simulink model "SEPIC_hybrid_closed_loop"  (R2020a)
settings: Solver=FixedStepAuto  StartTime=0.0  StopTime=0.05  FixedStep=Ts  RelTol=1e-8
values from neighbouring files (symbols this model uses):
  E = 300    [parameters_SEPIC.m]    (also in test_sepic_1.m = @(t) 300)
  L1 = 2.57e-3    (= 0.00257)    [parameters_SEPIC.m]
  L2 = 1.71e-3    (= 0.00171)    [parameters_SEPIC.m]
  R = 80    [parameters_SEPIC.m]    (also in test_boost_1.m = @(t) (t <= tfin/2)*12 + (t>tfin/2)*15; test_sepic_1.m = @(t) 80)
  rC1 = 350e-3    (= 0.35)    [parameters_SEPIC.m]
  rC2 = 270e-3    (= 0.27)    [parameters_SEPIC.m]
  rDS1 = 0.01    [parameters_SEPIC.m]
  rDS2 = 80e-3    (= 0.08)    [parameters_SEPIC.m]
  Ts = 1/fPWM/100    (= 1e-07)    [parameters_SEPIC.m]
  VF1 = 0.2    [parameters_SEPIC.m]
  VF2 = 0.62    [parameters_SEPIC.m]
undefined symbols (not defined in the file or in its folder): Down, Ks, Up
libraries: fl_lib x13, nesl_utility x12, ee_lib x4, simulink x2, eePwmGenerator x1
settings Model: Creator=Vlad  LastModifiedBy=mircea
settings SFSimCC: CustomCodeUndefinedFunction=UseInterfaceOnly

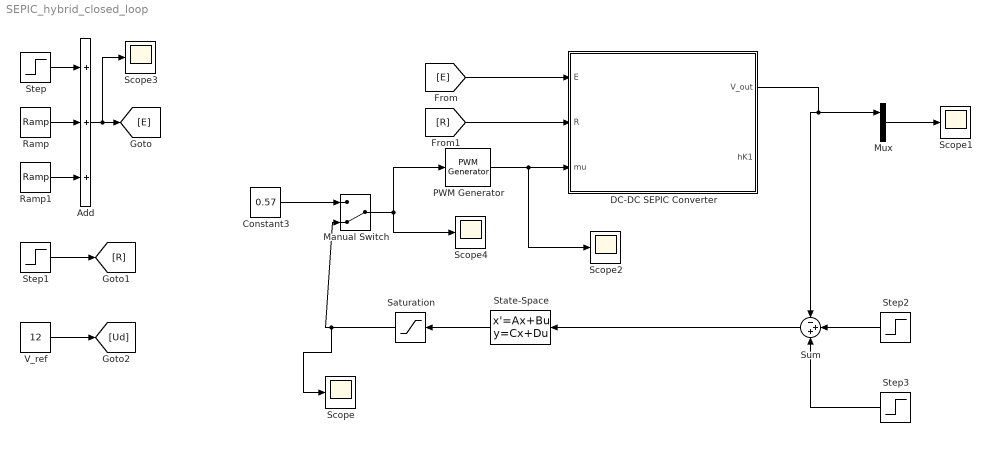
== system SEPIC_hybrid_closed_loop ==
  Add : Sum  Inputs=+++
  Constant3 : Constant  Value=0.57
  DC-DC SEPIC Converter : Subsystem
  Manual Switch : ManualSwitch  CurrentSetting=0
  Mux : Mux  Inputs=2
  PWM Generator : eePwmGenerator/PWM Generator  CarrCount=Up-Down  Tper=TPWM  Ts=Ts
  Ramp : simulink/Sources/Ramp  slope=30  start=0.2  InitialOutput=0
  Ramp1 : simulink/Sources/Ramp  slope=-60  start=0.3  InitialOutput=0
  Saturation : Saturate  UpperLimit=0.95  LowerLimit=0
  Scope{,1..4} (5 alike) : Scope
  State-Space : StateSpace  A=Ks.A  B=Ks.B  C=Ks.C  D=Ks.D  InitialCondition=0
  Step : Step  Time=0.1  Before=E  After=1.2*E  SampleTime=0
  Step1 : Step  Time=0.15  Before=R  After=1.2*R  SampleTime=0
  Step2 : Step  Time=0.01  Before=380  After=400  SampleTime=0
  Step3 : Step  Time=0.025  After=20  SampleTime=0
  Sum : Sum  Inputs=-++
  V_ref : Constant  Value=12
  wires:
  V_ref/1 -> [Ud]
  Step1/1 -> [R]
  Ramp1/1 -> Add/3
  Ramp/1 -> Add/2
  Step/1 -> Add/1
  Add/1 -> Scope3/1, [E]
  [R] -> DC-DC SEPIC Converter/2(R)
  [E] -> DC-DC SEPIC Converter/1(E)
  Constant3/1 -> Manual Switch/1
  Manual Switch/1 -> Scope4/1, PWM Generator/1
  Mux/1 -> Scope1/1
  DC-DC SEPIC Converter/1(V_out) -> Sum/1, Mux/1
  PWM Generator/1 -> Scope2/1, DC-DC SEPIC Converter/3(mu)
  Step2/1 -> Sum/2
  Sum/1 -> State-Space/1
  State-Space/1 -> Saturation/1
  Saturation/1 -> Scope/1, Manual Switch/2
  Step3/1 -> Sum/3

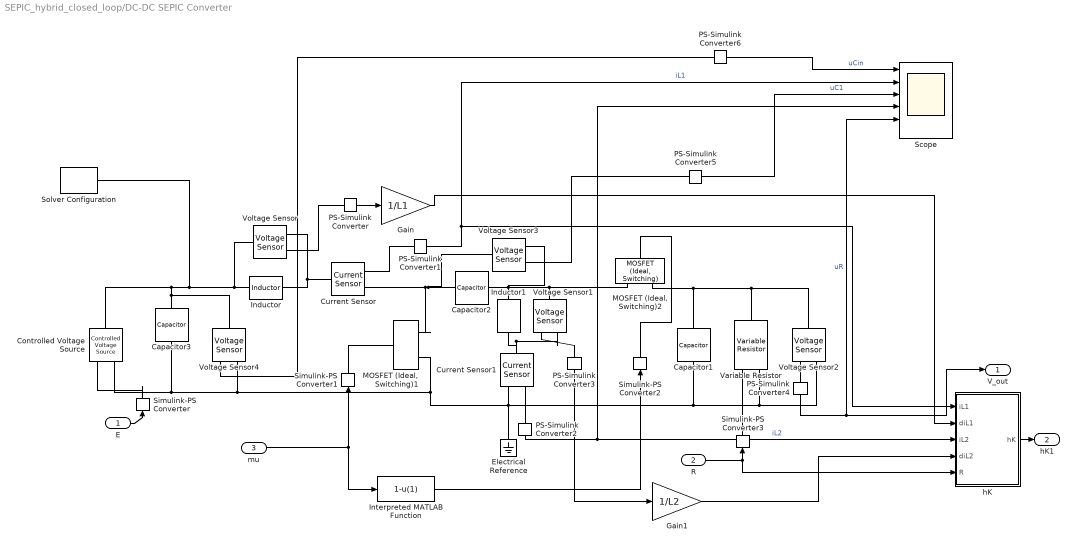
== system SEPIC_hybrid_closed_loop/DC-DC SEPIC Converter ==
  E : Inport
  R : Inport  Port=2
  mu : Inport  Port=3
  Capacitor1 : fl_lib/Electrical/Electrical Elements/Capacitor  c=C2 F  r=rC2 Ohm  g=0 1/Ohm  i_specify=off  i_priority=None  i=0 A  i_nominal_specify=off  i_nominal_unit=A  i_nominal_value=1  v_specify=on  v_priority=None  v=uC20 V  v_nominal_specify=off  v_nominal_unit=V  v_nominal_value=1  vc_specify=off  vc_priority=High  vc=0 V  vc_nominal_specify=off  vc_nominal_unit=V  vc_nominal_value=1
  Capacitor2 : fl_lib/Electrical/Electrical Elements/Capacitor  c=C1 F  r=rC1 Ohm  g=0 1/Ohm  i_specify=off  i_priority=None  i=0 A  i_nominal_specify=off  i_nominal_unit=A  i_nominal_value=1  v_specify=on  v_priority=None  v=uC10 V  v_nominal_specify=off  v_nominal_unit=V  v_nominal_value=1  vc_specify=off  vc_priority=High  vc=0 V  vc_nominal_specify=off  vc_nominal_unit=V  vc_nominal_value=1
  Capacitor3 : fl_lib/Electrical/Electrical Elements/Capacitor  c=Cin F  r=rCin Ohm  g=0 1/Ohm  i_specify=off  i_priority=None  i=0 A  i_nominal_specify=off  i_nominal_unit=A  i_nominal_value=1  v_specify=on  v_priority=None  v=uCin0 V  v_nominal_specify=off  v_nominal_unit=V  v_nominal_value=1  vc_specify=off  vc_priority=High  vc=0 V  vc_nominal_specify=off  vc_nominal_unit=V  vc_nominal_value=1
  Controlled Voltage Source : fl_lib/Electrical/Electrical Sources/Controlled Voltage Source
  Current Sensor : fl_lib/Electrical/Electrical Sensors/Current Sensor
  Current Sensor1 : fl_lib/Electrical/Electrical Sensors/Current Sensor
  Electrical Reference : fl_lib/Electrical/Electrical Elements/Electrical Reference
  Gain : Gain  Gain=1/L1
  Gain1 : Gain  Gain=1/L2
  Inductor : ee_lib/Passive/Inductor  l=L1 H  L_tol=20  enable_L_tol=0  tol_distribution=1  nSigma=4  r=rL1 Ohm  g=0 1/Ohm  enable_operating_limits=0  operating_limit_action=2  max_working_current=1 A  power_rating=1 W  enable_faults=0  fault_action=1  lambdaPercent=50  k_faulted=0.9999  turnsShort=0  openCct=0  groundShort=0  groundShortG=0 1/Ohm  tau_fault=1e-3 s  enable_temporal_fault=0  t_fault=1 s  enable_behavioral_fault=0  max_permissible_voltage=100 V  n_fail_on_voltage=1  max_permissible_current=1 A  t_fail_on_current=1 s  i_L_specify=on  i_L_priority=High  i_L=iL10 A  i_L_nominal_specify=off  i_L_nominal_unit=A  i_L_nominal_value=1
  Inductor1 : ee_lib/Passive/Inductor  l=L2 H  L_tol=20  enable_L_tol=0  tol_distribution=1  nSigma=4  r=rL2 Ohm  g=0 1/Ohm  enable_operating_limits=0  operating_limit_action=2  max_working_current=1 A  power_rating=1 W  enable_faults=0  fault_action=1  lambdaPercent=50  k_faulted=0.9999  turnsShort=0  openCct=0  groundShort=0  groundShortG=0 1/Ohm  tau_fault=1e-3 s  enable_temporal_fault=0  t_fault=1 s  enable_behavioral_fault=0  max_permissible_voltage=100 V  n_fail_on_voltage=1  max_permissible_current=1 A  t_fail_on_current=1 s  i_L_specify=on  i_L_priority=High  i_L=iL20 A  i_L_nominal_specify=off  i_L_nominal_unit=A  i_L_nominal_value=1
  Interpreted MATLAB Function : MATLABFcn  MATLABFcn=1-u(1)
  "MOSFET (Ideal, Switching)1" : ee_lib/Semiconductors & Converters/MOSFET (Ideal, Switching)  Rds=rDS1 Ohm  Goff=1e-6 1/Ohm  Vth=0.5 V  diode_param=2  diode_Vf=VF1 V  diode_Ron=0.001 Ohm  diode_Goff=1e-5 1/Ohm  diode_C=50e-9 F  diode_iRM=-235 A  diode_iF=300 A  diode_idot=-50 A/us  diode_trr_param=1  diode_trr_factor=3  diode_trr=15 us  diode_Qrr=1500 s*uA  thermal_loss_option=ee.enum.converters.thermalLossOption.constantvalues  Voff=300 V  Tau=1e-4 s  Tj=[298.15, 398.15] K  Iout_scalar=600 A  Eon_scalar=22.86e-3 J  Eoff_scalar=17.14e-3 J  Von_scalar=2.7 V  Iout_data=[0, 10, 50, 100, 200, 400, 600] A  Eon_data=[0, .29, 1.43, 2.86, 5.71, 13.14, 22.86; 0, .57, 2.63, 5.14, 10.29, 20.57, 30.29] * 1e-3 J  Eoff_data=[0, .21, 1.07, 2.14, 4.29, 9.86, 17.14; 0, .43, 1.97, 3.86, 7.71, 15.43, 22.71] * 1e-3 J  Von_data=[0, 1.1, 1.3, 1.45, 1.75, 2.25, 2.7; 0, 1, 1.15, 1.35, 1.7, 2.35, 3] V
  "MOSFET (Ideal, Switching)2" : ee_lib/Semiconductors & Converters/MOSFET (Ideal, Switching)  Rds=rDS2 Ohm  Goff=1e-6 1/Ohm  Vth=0.5 V  diode_param=2  diode_Vf=VF2 V  diode_Ron=0.001 Ohm  diode_Goff=1e-5 1/Ohm  diode_C=50e-9 F  diode_iRM=-235 A  diode_iF=300 A  diode_idot=-50 A/us  diode_trr_param=1  diode_trr_factor=3  diode_trr=15 us  diode_Qrr=1500 s*uA  thermal_loss_option=ee.enum.converters.thermalLossOption.constantvalues  Voff=300 V  Tau=1e-4 s  Tj=[298.15, 398.15] K  Iout_scalar=600 A  Eon_scalar=22.86e-3 J  Eoff_scalar=17.14e-3 J  Von_scalar=2.7 V  Iout_data=[0, 10, 50, 100, 200, 400, 600] A  Eon_data=[0, .29, 1.43, 2.86, 5.71, 13.14, 22.86; 0, .57, 2.63, 5.14, 10.29, 20.57, 30.29] * 1e-3 J  Eoff_data=[0, .21, 1.07, 2.14, 4.29, 9.86, 17.14; 0, .43, 1.97, 3.86, 7.71, 15.43, 22.71] * 1e-3 J  Von_data=[0, 1.1, 1.3, 1.45, 1.75, 2.25, 2.7; 0, 1, 1.15, 1.35, 1.7, 2.35, 3] V
  PS-Simulink Converter{,1..6} (7 alike) : nesl_utility/PS-Simulink Converter  PhysicalDomain=network_engine_domain  SubClassName=ps_output  LeftPortType=input  RightPortType=output  PseudoPeriodic=off  Frequencies=[]  Unit=inherit  AffineConversion=off
  Scope : Scope  NumInputPorts=6
  Simulink-PS Converter{,1..3} (4 alike) : nesl_utility/Simulink-PS Converter  PhysicalDomain=network_engine_domain  SubClassName=ps_input  LeftPortType=input  RightPortType=output  PseudoPeriodic=off  Frequencies=[]  NoiseDistribution=none  NoiseParameters=[]  Unit=1  AffineConversion=off  FilteringAndDerivatives=provide  SimscapeFilterOrder=1  InputFilterTimeConstant=0.001  UdotUserProvided=0
  Solver Configuration : nesl_utility/Solver Configuration  PhysicalDomain=network_engine_domain  SubClassName=solver  LeftPortType=input  RightPortType=generic  Tones=[]  Harmonics=[]  SimulateNoise=off  Profile=off  UseLocalSampling=off  EnableSwitchedLinearOptims=on  FrequencyDomain=off  UseCCode=off  RelTol=0.001  AbsTol=1e-06  MinStep=1e-09  ToWorkspace=off  RevertToSquareIcSolve=off  NumHomotopyIterations=100  PhasorMode=off  PhasorModeNumHarmonics=1  DoDC=off  ResidualTolerance=1e-09  UseLocalSolver=on  LocalSolverChoice=NE_TRAPEZOIDAL_ADVANCER  LocalSolverSampleTime=Ts  DoFixedCost=off  MaxNonlinIter=3  MaxModeIter=2  LinearAlgebra=auto  EquationFormulation=NE_TIME_EF  DelaysMemoryBudget=1024  AutomaticFiltering=on  FilteringTimeConstant=0.001  PartitionStorageMethod=AS_NEEDED  PartitionMemoryBudget=1024  PartitionMethod=ROBUST
  Variable Resistor : fl_lib/Electrical/Electrical Elements/Variable Resistor  Rmin=0 Ohm  i_specify=off  i_priority=None  i=0 A  i_nominal_specify=off  i_nominal_unit=A  i_nominal_value=1  v_specify=off  v_priority=None  v=0 V  v_nominal_specify=off  v_nominal_unit=V  v_nominal_value=1
  Voltage Sensor{,1..4} (5 alike) : fl_lib/Electrical/Electrical Sensors/Voltage Sensor
  hK : Subsystem
  V_out : Outport
  hK1 : Outport  Port=2
  wires:
  E/1 -> Simulink-PS Converter/1
  Interpreted MATLAB Function/1 -> Simulink-PS Converter2/1
  Gain1/1 -> hK/4(diL2)
  PS-Simulink Converter2/1 -> Scope/4, hK/3(iL2)  "iL2"
  PS-Simulink Converter/1 -> Gain/1
  Gain/1 -> hK/2(diL1)
  R/1 -> hK/5(R), Simulink-PS Converter3/1
  PS-Simulink Converter3/1 -> Gain1/1
  PS-Simulink Converter1/1 -> Scope/2, hK/1(iL1)  "iL1"
  mu/1 -> Simulink-PS Converter1/1, Interpreted MATLAB Function/1
  PS-Simulink Converter4/1 -> Scope/5, V_out/1  "uR"
  hK/1(hK) -> hK1/1
  PS-Simulink Converter5/1 -> Scope/3  "uC1"
  PS-Simulink Converter6/1 -> Scope/1  "uCin"
  connections:
  Inductor1/LConn1 -- Voltage Sensor3/RConn2 -- "MOSFET (Ideal, Switching)2"/RConn2 -- Voltage Sensor1/LConn1 -- Capacitor2/RConn1
  Controlled Voltage Source/LConn1 -- Voltage Sensor4/LConn1 -- Capacitor3/LConn1 -- Solver Configuration/RConn1 -- Voltage Sensor/LConn1 -- Inductor/LConn1
  PS-Simulink Converter4/LConn1 -- Voltage Sensor2/RConn1
  Current Sensor1/LConn1 -- Voltage Sensor1/RConn2 -- Inductor1/RConn1
  Current Sensor/LConn1 -- Voltage Sensor/RConn2 -- Inductor/RConn1
  Capacitor1/LConn1 -- "MOSFET (Ideal, Switching)2"/RConn1 -- Voltage Sensor2/LConn1 -- Variable Resistor/RConn1
  Electrical Reference/LConn1 -- Capacitor3/RConn1 -- Controlled Voltage Source/RConn2 -- Voltage Sensor4/RConn2 -- "MOSFET (Ideal, Switching)1"/RConn2 -- Current Sensor1/RConn2 -- Capacitor1/RConn1 -- Variable Resistor/LConn2 -- Voltage Sensor2/RConn2
  PS-Simulink Converter3/LConn1 -- Voltage Sensor1/RConn1
  PS-Simulink Converter1/LConn1 -- Current Sensor/RConn1
  PS-Simulink Converter2/LConn1 -- Current Sensor1/RConn1
  PS-Simulink Converter/LConn1 -- Voltage Sensor/RConn1
  Simulink-PS Converter3/RConn1 -- Variable Resistor/LConn1
  "MOSFET (Ideal, Switching)1"/RConn1 -- Voltage Sensor3/LConn1 -- Capacitor2/LConn1 -- Current Sensor/RConn2
  Simulink-PS Converter2/RConn1 -- "MOSFET (Ideal, Switching)2"/LConn1
  Simulink-PS Converter1/RConn1 -- "MOSFET (Ideal, Switching)1"/LConn1
  Simulink-PS Converter/RConn1 -- Controlled Voltage Source/RConn1
  Voltage Sensor3/RConn1 -- PS-Simulink Converter5/LConn1
  PS-Simulink Converter6/LConn1 -- Voltage Sensor4/RConn1

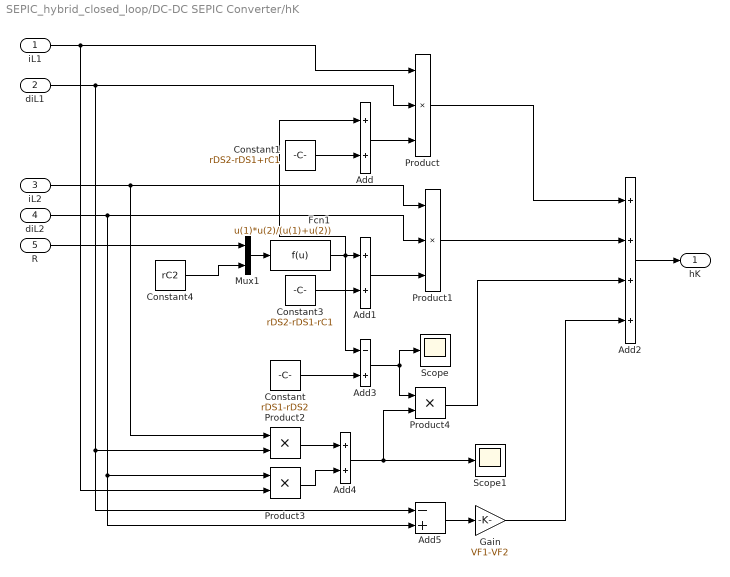
== system SEPIC_hybrid_closed_loop/DC-DC SEPIC Converter/hK ==
  iL1 : Inport
  diL1 : Inport  Port=2
  iL2 : Inport  Port=3
  diL2 : Inport  Port=4
  R : Inport  Port=5
  Add : Sum
  Add1 : Sum
  Add2 : Sum  Inputs=++++
  Add3 : Sum  Inputs=-+
  Add4 : Sum
  Add5 : Sum  Inputs=-+
  Constant : Constant  Value=rDS1-rDS2
  Constant1 : Constant  Value=rDS2-rDS1+rC1
  Constant3 : Constant  Value=rDS2-rDS1-rC1
  Constant4 : Constant  Value=rC2
  Fcn1 : Fcn  Expr=u(1)*u(2)/(u(1)+u(2))
  Gain : Gain  Gain=VF1-VF2
  Mux1 : Mux  Inputs=2
  Product : Product  Inputs=3
  Product1 : Product  Inputs=3
  Product2 : Product
  Product3 : Product
  Product4 : Product
  Scope : Scope
  Scope1 : Scope
  hK : Outport  VectorParamsAs1DForOutWhenUnconnected=off
  wires:
  Add1/1 -> Product1/3
  Add/1 -> Product/3
  Constant3/1 -> Add1/2
  diL2/1 -> Add5/2, Product3/1, Product1/2
  Fcn1/1 -> Add3/1, Add/1, Add1/1
  Product1/1 -> Add2/2
  Mux1/1 -> Fcn1/1
  diL1/1 -> Add5/1, Product2/2, Product/2
  Constant4/1 -> Mux1/2
  Constant1/1 -> Add/2
  iL2/1 -> Product2/1, Product1/1
  iL1/1 -> Product3/2, Product/1
  R/1 -> Mux1/1
  Add2/1 -> hK/1
  Product/1 -> Add2/1
  Constant/1 -> Add3/2
  Product2/1 -> Add4/1
  Product3/1 -> Add4/2
  Add3/1 -> Product4/1, Scope/1
  Product4/1 -> Add2/3
  Add5/1 -> Gain/1
  Gain/1 -> Add2/4
  Add4/1 -> Product4/2, Scope1/1
